simulink model "snb_bcxx"  (R2012b)
settings: Solver=FixedStepDiscrete  SolverMode=SingleTasking  StartTime=0.0  StopTime=10000  RelTol=1e-3
undefined symbols (not defined in the file): Down, pfb_coeff_gen_calc, Up
libraries: xbsIndex_r4 x19669, casper_library_misc x44, casper_library_delays x18, casper_library_communications x8, xps_library x3
(part 13 of 159)

== system snb_bcxx/pack ==
  note: Prevent transmission of data
      | before we have seen the first
      | sync
  rst : Inport
  sync_in : Inport  Port=2
  en : Inport  Port=3
  din : Inport  Port=4
  timestamp : Inport  Port=5
  flag : Inport  Port=6
  board_id : Inport  Port=7
  base_ip : Inport  Port=8
  base_port : Inport  Port=9
  AddSub : xbsIndex_r4/AddSub  mode=Addition  use_carryin=off  use_carryout=off  en=off  latency=1  precision=User Defined  arith_type=Unsigned  n_bits=32  bin_pt=0  quantization=Truncate  overflow=Wrap  dbl_ovrd=off  use_behavioral_HDL=off  hw_selection=Fabric  pipelined=off  block_type=addsub
  AddSub1 : xbsIndex_r4/AddSub  mode=Subtraction  use_carryin=off  use_carryout=off  en=on  latency=1  precision=Full  arith_type=Unsigned  n_bits=16  bin_pt=14  quantization=Truncate  overflow=Wrap  dbl_ovrd=off  use_behavioral_HDL=off  hw_selection=Fabric  pipelined=off  block_type=addsub
  Concat{,1..4} (5 alike) : xbsIndex_r4/Concat  num_inputs=2  dbl_ovrd=off  block_type=concat
  Concat10 : xbsIndex_r4/Concat  num_inputs=3  dbl_ovrd=off  block_type=concat
  Concat{5..8} (4 alike) : xbsIndex_r4/Concat  num_inputs=4  dbl_ovrd=off  block_type=concat
  Concat9 : xbsIndex_r4/Concat  num_inputs=3  dbl_ovrd=off  block_type=concat
  Constant : xbsIndex_r4/Constant  const=0  gui_display_data_type=Fixed-point  arith_type=Unsigned  n_bits=n_bits_packet - n_bits_inputs  bin_pt=0  preci_type=Single  exp_width=8  frac_width=24  explicit_period=on  period=1  equ=P=C  opselect=C  inp2=PCIN>>17  opr=+  inp1=P  carry=CIN  dbl_ovrd=off  block_type=constant
  Constant1 : xbsIndex_r4/Constant  const=0  gui_display_data_type=Fixed-point  arith_type=Unsigned  n_bits=2  bin_pt=0  preci_type=Single  exp_width=8  frac_width=24  explicit_period=on  period=1  equ=P=C  opselect=C  inp2=PCIN>>17  opr=+  inp1=P  carry=CIN  dbl_ovrd=off  block_type=constant
  Constant{7,10,13,16..19,39} (8 alike) : xbsIndex_r4/Constant  const=0  gui_display_data_type=Fixed-point  arith_type=Unsigned  n_bits=48  bin_pt=0  preci_type=Single  exp_width=8  frac_width=24  explicit_period=on  period=1  equ=P=C  opselect=C  inp2=PCIN>>17  opr=+  inp1=P  carry=CIN  dbl_ovrd=off  block_type=constant
  Constant{5,8,11,14} (4 alike) : xbsIndex_r4/Constant  const=1  gui_display_data_type=Fixed-point  arith_type=Unsigned  n_bits=48  bin_pt=0  preci_type=Single  exp_width=8  frac_width=24  explicit_period=on  period=1  equ=P=C  opselect=C  inp2=PCIN>>17  opr=+  inp1=P  carry=CIN  dbl_ovrd=off  block_type=constant
  Constant{6,9,12,15} (4 alike) : xbsIndex_r4/Constant  const=2^(n_bits_packet-n_bits_inputs)  gui_display_data_type=Fixed-point  arith_type=Unsigned  n_bits=48  bin_pt=0  preci_type=Single  exp_width=8  frac_width=24  explicit_period=on  period=1  equ=P=C  opselect=C  inp2=PCIN>>17  opr=+  inp1=P  carry=CIN  dbl_ovrd=off  block_type=constant
  Constant2 : xbsIndex_r4/Constant  const=1  gui_display_data_type=Fixed-point  arith_type=Unsigned  n_bits=2  bin_pt=0  preci_type=Single  exp_width=8  frac_width=24  explicit_period=on  period=1  equ=P=C  opselect=C  inp2=PCIN>>17  opr=+  inp1=P  carry=CIN  dbl_ovrd=off  block_type=constant
  Constant20 : xbsIndex_r4/Constant  const=0  gui_display_data_type=Fixed-point  arith_type=Unsigned  n_bits=n_bits_frequencies + n_bits_packet - n_bits_inputs  bin_pt=0  preci_type=Single  exp_width=8  frac_width=24  explicit_period=on  period=1  equ=P=C  opselect=C  inp2=PCIN>>17  opr=+  inp1=P  carry=CIN  dbl_ovrd=off  block_type=constant
  Constant3 : xbsIndex_r4/Constant  const=2  gui_display_data_type=Fixed-point  arith_type=Unsigned  n_bits=2  bin_pt=0  preci_type=Single  exp_width=8  frac_width=24  explicit_period=on  period=1  equ=P=C  opselect=C  inp2=PCIN>>17  opr=+  inp1=P  carry=CIN  dbl_ovrd=off  block_type=constant
  Constant4 : xbsIndex_r4/Constant  const=3  gui_display_data_type=Fixed-point  arith_type=Unsigned  n_bits=2  bin_pt=0  preci_type=Single  exp_width=8  frac_width=24  explicit_period=on  period=1  equ=P=C  opselect=C  inp2=PCIN>>17  opr=+  inp1=P  carry=CIN  dbl_ovrd=off  block_type=constant
  Convert{,2..9} (9 alike) : xbsIndex_r4/Convert  gui_display_data_type=Fixed-point  arith_type=Unsigned  n_bits=48  bin_pt=0  float_type=Single  exp_bits=8  fraction_bits=24  quantization=Truncate  overflow=Wrap  en=off  latency=0  dbl_ovrd=off  pipeline=off  block_type=convert
  Convert10 : xbsIndex_r4/Convert  gui_display_data_type=Fixed-point  arith_type=Unsigned  n_bits=32  bin_pt=0  float_type=Single  exp_bits=8  fraction_bits=24  quantization=Truncate  overflow=Wrap  en=off  latency=0  dbl_ovrd=off  pipeline=off  block_type=convert
  Delay{,16..20,27,31,33..34,37,39} (12 alike) : xbsIndex_r4/Delay  rst=off  infoeditControl=Selection of Reset will increase slice count due to use of real FFs and instead of SRLs  en=off  latency=1  dbl_ovrd=off  reg_retiming=on  block_type=delay
  Delay{1..15,21..26,28..30,32,35..36} (27 alike) : xbsIndex_r4/Delay  rst=off  infoeditControl=Selection of Reset will increase slice count due to use of real FFs and instead of SRLs  en=off  latency=2  dbl_ovrd=off  reg_retiming=on  block_type=delay
  Delay38 : xbsIndex_r4/Delay  rst=off  infoeditControl=Selection of Reset will increase slice count due to use of real FFs and instead of SRLs  en=off  latency=1  dbl_ovrd=off  reg_retiming=off  block_type=delay
  Logical{,1,6..8} (5 alike) : xbsIndex_r4/Logical  logical_function=AND  inputs=2  en=off  latency=0  precision=Full  arith_type=Unsigned  n_bits=16  bin_pt=0  align_bp=on  dbl_ovrd=off  block_type=logical
  Logical{2..5} (4 alike) : xbsIndex_r4/Logical  logical_function=AND  inputs=2  en=off  latency=1  precision=Full  arith_type=Unsigned  n_bits=16  bin_pt=0  align_bp=on  dbl_ovrd=off  block_type=logical
  Register : xbsIndex_r4/Register  init=0  rst=on  en=on  dbl_ovrd=off  block_type=register
  Register1 : xbsIndex_r4/Register  init=0  rst=on  en=on  dbl_ovrd=off  block_type=register
  Relational : xbsIndex_r4/Relational  mode=a=b  en=off  latency=0  dbl_ovrd=off  block_type=relational
  Relational1 : xbsIndex_r4/Relational  mode=a=b  en=off  latency=0  dbl_ovrd=off  block_type=relational
  Relational2 : xbsIndex_r4/Relational  mode=a!=b  en=off  latency=1  dbl_ovrd=off  block_type=relational
  Relational3 : xbsIndex_r4/Relational  mode=a!=b  en=off  latency=1  dbl_ovrd=off  block_type=relational
  Slice1 : xbsIndex_r4/Slice  nbits=n_bits_xengines - n_bits_xeng_per_ip  boolean_output=off  mode=Upper Bit Location + Width  bit1=0  base1=MSB of Input  bit0=0  base0=LSB of Input  dbl_ovrd=off  block_type=slice
  Slice2 : xbsIndex_r4/Slice  nbits=48  boolean_output=off  mode=Upper Bit Location + Width  bit1=0  base1=MSB of Input  bit0=0  base0=LSB of Input  dbl_ovrd=off  block_type=slice
  Slice3 : xbsIndex_r4/Slice  nbits=48  boolean_output=off  mode=Two Bit Locations  bit1=0  base1=MSB of Input  bit0=9+3  base0=LSB of Input  dbl_ovrd=off  block_type=slice
  Slice4 : xbsIndex_r4/Slice  nbits=4  boolean_output=off  mode=Lower Bit Location + Width  bit1=0  base1=MSB of Input  bit0=0  base0=LSB of Input  dbl_ovrd=off  block_type=slice
  Slice5 : xbsIndex_r4/Slice  nbits=48  boolean_output=off  mode=Two Bit Locations  bit1=0  base1=MSB of Input  bit0=9+3  base0=LSB of Input  dbl_ovrd=off  block_type=slice
  Slice6 : xbsIndex_r4/Slice  nbits=12  boolean_output=off  mode=Lower Bit Location + Width  bit1=0  base1=MSB of Input  bit0=0  base0=LSB of Input  dbl_ovrd=off  block_type=slice
  Terminator{15..18} (4 alike) : Terminator
  bus_expand : Subsystem  AncestorBlock=casper_library_flow_control/bus_expand  mask(bus_expand){mode=divisions of equal size, outputNum=4, outputWidth=64, outputBinaryPt=0, outputArithmeticType=0, show_format=off, outputToWorkspace=off, variablePrefix=out, outputToModelAsWell=on}
      mask prompts: outputNum "Number of outputs:"; outputWidth "Output width:"; outputBinaryPt "Output binary point position:"; outputArithmeticType "Output arithmetic type (ufix=0, fix=1, bool=2):"; show_format "Print format string?"; outputToWorkspace "Output to workspace?"; variablePrefix "Variable name prefix:"; outputToModelAsWell "Output to model as well?"
      mask help:
      | Expands a 'bus' made using a bus_create or Xilinx
      | concat block.
      | The input will be divided into the specified number
      | of outputs with the specified arithmetic types.
      | Divisions are made from most significant bit.
      mask init: same as snb_bcxx/bus_expand10
      settings: AttributesFormatString=4 outputs
      mask TypeOptions mode: divisions of equal size | divisions of arbitrary size
      mask Callback mode: bus_expand_callback();
      mask Callback outputWidth: bus_expand_callback();
      mask Callback outputToWorkspace: bus_expand_callback();
  bus_expand1 : Subsystem  AncestorBlock=casper_library_flow_control/bus_expand  mask(bus_expand){mode=divisions of equal size, outputNum=4, outputWidth=1, outputBinaryPt=0, outputArithmeticType=0, show_format=off, outputToWorkspace=off, variablePrefix=out, outputToModelAsWell=on}
      mask prompts: outputNum "Number of outputs:"; outputWidth "Output width:"; outputBinaryPt "Output binary point position:"; outputArithmeticType "Output arithmetic type (ufix=0, fix=1, bool=2):"; show_format "Print format string?"; outputToWorkspace "Output to workspace?"; variablePrefix "Variable name prefix:"; outputToModelAsWell "Output to model as well?"
      mask help:
      | Expands a 'bus' made using a bus_create or Xilinx
      | concat block.
      | The input will be divided into the specified number
      | of outputs with the specified arithmetic types.
      | Divisions are made from most significant bit.
      mask init: same as snb_bcxx/bus_expand10
      settings: AttributesFormatString=4 outputs
      mask TypeOptions mode: divisions of equal size | divisions of arbitrary size
      mask Callback mode: bus_expand_callback();
      mask Callback outputWidth: bus_expand_callback();
      mask Callback outputToWorkspace: bus_expand_callback();
  bus_expand2 : Subsystem  AncestorBlock=casper_library_flow_control/bus_expand  mask(bus_expand){mode=divisions of equal size, outputNum=4, outputWidth=16, outputBinaryPt=0, outputArithmeticType=0, show_format=off, outputToWorkspace=off, variablePrefix=out, outputToModelAsWell=on}
      mask prompts: outputNum "Number of outputs:"; outputWidth "Output width:"; outputBinaryPt "Output binary point position:"; outputArithmeticType "Output arithmetic type (ufix=0, fix=1, bool=2):"; show_format "Print format string?"; outputToWorkspace "Output to workspace?"; variablePrefix "Variable name prefix:"; outputToModelAsWell "Output to model as well?"
      mask help:
      | Expands a 'bus' made using a bus_create or Xilinx
      | concat block.
      | The input will be divided into the specified number
      | of outputs with the specified arithmetic types.
      | Divisions are made from most significant bit.
      mask init: same as snb_bcxx/bus_expand10
      settings: AttributesFormatString=4 outputs
      mask TypeOptions mode: divisions of equal size | divisions of arbitrary size
      mask Callback mode: bus_expand_callback();
      mask Callback outputWidth: bus_expand_callback();
      mask Callback outputToWorkspace: bus_expand_callback();
  count : xbsIndex_r4/Counter  cnt_type=Free Running  cnt_to=Inf  operation=Up  start_count=0  cnt_by_val=1  arith_type=Unsigned  n_bits=n_bits_frequencies + n_bits_packet - n_bits_inputs  bin_pt=0  load_pin=off  rst=on  en=on  explicit_period=on  period=1  dbl_ovrd=off  use_behavioral_HDL=off  implementation=Fabric  block_type=counter
  count1 : xbsIndex_r4/Counter  cnt_type=Free Running  cnt_to=Inf  operation=Up  start_count=0  cnt_by_val=1  arith_type=Unsigned  n_bits=n_bits_xengines  bin_pt=0  load_pin=off  rst=on  en=on  explicit_period=on  period=1  dbl_ovrd=off  use_behavioral_HDL=off  implementation=Fabric  block_type=counter
  divisions : xbsIndex_r4/Slice  nbits=n_bits_frequencies - n_bits_xengines  boolean_output=off  mode=Upper Bit Location + Width  bit1=0  base1=MSB of Input  bit0=0  base0=LSB of Input  dbl_ovrd=off  block_type=slice
  expected_diff : xbsIndex_r4/Constant  const=2^9  gui_display_data_type=Fixed-point  arith_type=Unsigned  n_bits=10  bin_pt=0  preci_type=Single  exp_width=8  frac_width=24  explicit_period=on  period=1  equ=P=C  opselect=C  inp2=PCIN>>17  opr=+  inp1=P  carry=CIN  dbl_ovrd=off  block_type=constant
  frequency : xbsIndex_r4/Slice  nbits=n_bits_frequencies  boolean_output=off  mode=Upper Bit Location + Width  bit1=0  base1=MSB of Input  bit0=0  base0=LSB of Input  dbl_ovrd=off  block_type=slice
  hdra_5 : xbsIndex_r4/Assert  assert_type=on  type_source=Explicitly  gui_display_data_type=Fixed-point  arith_type=Unsigned  n_bits=48  bin_pt=0  preci_type=Single  exp_width=8  frac_width=24  assert_rate=off  rate_source=Explicitly  period=1  output_port=on  block_type=assert
  pipeline1 : Subsystem  AncestorBlock=casper_library_delays/pipeline  mask(pipeline){latency=2}
      mask help:
      | An explicitly laid-out delay line to avoid mapping to SRL16s
      | for use in pipelining to help achieve timing closure.
      mask init:
      | pipeline_init(gcb,'latency',latency);
      settings: AttributesFormatString=Latency = %<latency>
      mask Display:
      | port_label('input', 1, 'd');
      | port_label('output', 1, 'q');
      | disp(['Z^-', num2str(latency)]);
  pipeline2 : Subsystem  AncestorBlock=casper_library_delays/pipeline  mask(pipeline){latency=1}
      mask help:
      | An explicitly laid-out delay line to avoid mapping to SRL16s
      | for use in pipelining to help achieve timing closure.
      mask init:
      | pipeline_init(gcb,'latency',latency);
      settings: AttributesFormatString=Latency = %<latency>
      mask Display:
      | port_label('input', 1, 'd');
      | port_label('output', 1, 'q');
      | disp(['Z^-', num2str(latency)]);
  pipeline3 : Subsystem  AncestorBlock=casper_library_delays/pipeline  mask(pipeline){latency=2}
      mask help:
      | An explicitly laid-out delay line to avoid mapping to SRL16s
      | for use in pipelining to help achieve timing closure.
      mask init:
      | pipeline_init(gcb,'latency',latency);
      settings: AttributesFormatString=Latency = %<latency>
      mask Display:
      | port_label('input', 1, 'd');
      | port_label('output', 1, 'q');
      | disp(['Z^-', num2str(latency)]);
  pipeline4 : Subsystem  AncestorBlock=casper_library_delays/pipeline  mask(pipeline){latency=2}
      mask help:
      | An explicitly laid-out delay line to avoid mapping to SRL16s
      | for use in pipelining to help achieve timing closure.
      mask init:
      | pipeline_init(gcb,'latency',latency);
      settings: AttributesFormatString=Latency = %<latency>
      mask Display:
      | port_label('input', 1, 'd');
      | port_label('output', 1, 'q');
      | disp(['Z^-', num2str(latency)]);
  pipeline5 : Subsystem  AncestorBlock=casper_library_delays/pipeline  mask(pipeline){latency=2}
      mask help:
      | An explicitly laid-out delay line to avoid mapping to SRL16s
      | for use in pipelining to help achieve timing closure.
      mask init:
      | pipeline_init(gcb,'latency',latency);
      settings: AttributesFormatString=Latency = %<latency>
      mask Display:
      | port_label('input', 1, 'd');
      | port_label('output', 1, 'q');
      | disp(['Z^-', num2str(latency)]);
  pipeline50 : Subsystem  AncestorBlock=casper_library_delays/pipeline  mask(pipeline){latency=2}
      mask help:
      | An explicitly laid-out delay line to avoid mapping to SRL16s
      | for use in pipelining to help achieve timing closure.
      mask init:
      | pipeline_init(gcb,'latency',latency);
      settings: AttributesFormatString=Latency = %<latency>
      mask Display:
      | port_label('input', 1, 'd');
      | port_label('output', 1, 'q');
      | disp(['Z^-', num2str(latency)]);
  pipeline6 : Subsystem  AncestorBlock=casper_library_delays/pipeline  mask(pipeline){latency=2}
      mask help:
      | An explicitly laid-out delay line to avoid mapping to SRL16s
      | for use in pipelining to help achieve timing closure.
      mask init:
      | pipeline_init(gcb,'latency',latency);
      settings: AttributesFormatString=Latency = %<latency>
      mask Display:
      | port_label('input', 1, 'd');
      | port_label('output', 1, 'q');
      | disp(['Z^-', num2str(latency)]);
  pipeline7 : Subsystem  AncestorBlock=casper_library_delays/pipeline  mask(pipeline){latency=2}
      mask help:
      | An explicitly laid-out delay line to avoid mapping to SRL16s
      | for use in pipelining to help achieve timing closure.
      mask init:
      | pipeline_init(gcb,'latency',latency);
      settings: AttributesFormatString=Latency = %<latency>
      mask Display:
      | port_label('input', 1, 'd');
      | port_label('output', 1, 'q');
      | disp(['Z^-', num2str(latency)]);
  sample_count : xbsIndex_r4/Slice  nbits=n_bits_packet - n_bits_inputs  boolean_output=off  mode=Lower Bit Location + Width  bit1=0  base1=MSB of Input  bit0=0  base0=LSB of Input  dbl_ovrd=off  block_type=slice
  select_we : xbsIndex_r4/Mux  inputs=2  en=off  latency=0  precision=Full  arith_type=Unsigned  n_bits=16  bin_pt=14  quantization=Truncate  overflow=Wrap  dbl_ovrd=off  block_type=mux
  spead_pack : Subsystem  Tag=casper:spead_pack  AncestorBlock=casper_library_communications/spead_pack  mask(pkt_pack_mask){max_pkt_len_bits=10, header_ids=0x1600, 0x4101, 0x4102, 0x4103, header_ind_ids=0x4300, spead_msw=64, spead_lsw=48, spead_version=4, bytes_per_word=8}
      mask prompts: max_pkt_len_bits "Max pkt length, 2^? 64-bit words"; header_ids "SPEAD direct address IDs (decimal)"; header_ind_ids "SPEAD indirect address IDs (decimal)"; spead_msw "SPEAD Flavour (MSw)"; spead_lsw "SPEAD Flavour (LSw)"; spead_version "SPEAD version"; bytes_per_word "Word size, in bytes"
      mask help:
      | This block generates SPEAD-compliant packets from a datastream.
      |
      | Packets are created with a fixed header followed by a number of 64-bit items.
      |
      | Requires a 64-bit data stream.
      |
      | The data_ready signal is one cycle BEFORE valid data! Does not have to be with a valid signal either.
      mask init:
      | if floor(log2(bytes_per_word)) ~= log2(bytes_per_word)
      |     error('Bytes per word should be a power of two.');
      | end
      | 
      | spead_pack_init(gcb)
  spead_pack1 : Subsystem  Tag=casper:spead_pack  AncestorBlock=casper_library_communications/spead_pack  mask(pkt_pack_mask){max_pkt_len_bits=10, header_ids=0x1600, 0x4101, 0x4102, 0x4103, header_ind_ids=0x4300, spead_msw=64, spead_lsw=48, spead_version=4, bytes_per_word=8}
      mask prompts: max_pkt_len_bits "Max pkt length, 2^? 64-bit words"; header_ids "SPEAD direct address IDs (decimal)"; header_ind_ids "SPEAD indirect address IDs (decimal)"; spead_msw "SPEAD Flavour (MSw)"; spead_lsw "SPEAD Flavour (LSw)"; spead_version "SPEAD version"; bytes_per_word "Word size, in bytes"
      mask help:
      | This block generates SPEAD-compliant packets from a datastream.
      |
      | Packets are created with a fixed header followed by a number of 64-bit items.
      |
      | Requires a 64-bit data stream.
      |
      | The data_ready signal is one cycle BEFORE valid data! Does not have to be with a valid signal either.
      mask init:
      | if floor(log2(bytes_per_word)) ~= log2(bytes_per_word)
      |     error('Bytes per word should be a power of two.');
      | end
      | 
      | spead_pack_init(gcb)
  spead_pack2 : Subsystem  Tag=casper:spead_pack  AncestorBlock=casper_library_communications/spead_pack  mask(pkt_pack_mask){max_pkt_len_bits=10, header_ids=0x1600, 0x4101, 0x4102, 0x4103, header_ind_ids=0x4300, spead_msw=64, spead_lsw=48, spead_version=4, bytes_per_word=8}
      mask prompts: max_pkt_len_bits "Max pkt length, 2^? 64-bit words"; header_ids "SPEAD direct address IDs (decimal)"; header_ind_ids "SPEAD indirect address IDs (decimal)"; spead_msw "SPEAD Flavour (MSw)"; spead_lsw "SPEAD Flavour (LSw)"; spead_version "SPEAD version"; bytes_per_word "Word size, in bytes"
      mask help:
      | This block generates SPEAD-compliant packets from a datastream.
      |
      | Packets are created with a fixed header followed by a number of 64-bit items.
      |
      | Requires a 64-bit data stream.
      |
      | The data_ready signal is one cycle BEFORE valid data! Does not have to be with a valid signal either.
      mask init:
      | if floor(log2(bytes_per_word)) ~= log2(bytes_per_word)
      |     error('Bytes per word should be a power of two.');
      | end
      | 
      | spead_pack_init(gcb)
  spead_pack3 : Subsystem  Tag=casper:spead_pack  AncestorBlock=casper_library_communications/spead_pack  mask(pkt_pack_mask){max_pkt_len_bits=10, header_ids=0x1600, 0x4101, 0x4102, 0x4103, header_ind_ids=0x4300, spead_msw=64, spead_lsw=48, spead_version=4, bytes_per_word=8}
      mask prompts: max_pkt_len_bits "Max pkt length, 2^? 64-bit words"; header_ids "SPEAD direct address IDs (decimal)"; header_ind_ids "SPEAD indirect address IDs (decimal)"; spead_msw "SPEAD Flavour (MSw)"; spead_lsw "SPEAD Flavour (LSw)"; spead_version "SPEAD version"; bytes_per_word "Word size, in bytes"
      mask help:
      | This block generates SPEAD-compliant packets from a datastream.
      |
      | Packets are created with a fixed header followed by a number of 64-bit items.
      |
      | Requires a 64-bit data stream.
      |
      | The data_ready signal is one cycle BEFORE valid data! Does not have to be with a valid signal either.
      mask init:
      | if floor(log2(bytes_per_word)) ~= log2(bytes_per_word)
      |     error('Bytes per word should be a power of two.');
      | end
      | 
      | spead_pack_init(gcb)
  wintime : xbsIndex_r4/Register  init=0  rst=off  en=on  dbl_ovrd=off  block_type=register
  wintime_old : xbsIndex_r4/Register  init=0  rst=off  en=on  dbl_ovrd=off  block_type=register
  xengines : xbsIndex_r4/Slice  nbits=n_bits_xengines  boolean_output=off  mode=Lower Bit Location + Width  bit1=0  base1=MSB of Input  bit0=0  base0=LSB of Input  dbl_ovrd=off  block_type=slice
  dout : Outport
  dvalid : Outport  Port=2
  eof : Outport  Port=3
  overflow : Outport  Port=4
  destination_ip : Outport  Port=5
  destination_port : Outport  Port=6
  wintime_snap : Outport  Port=7
  wintime_error : Outport  Port=8
  wintime_sp_error : Outport  Port=9
  wires:
  Slice1/1 -> Convert10/1
  Convert10/1 -> AddSub/2
  AddSub/1 -> destination_ip/1  "ip"
  count1/1 -> Slice1/1
  Delay19/1 -> destination_port/1  "port"
  base_port/1 -> Delay19/1
  Delay18/1 -> eof/1
  Delay16/1 -> dvalid/1
  Delay17/1 -> dout/1
  base_ip/1 -> AddSub/1
  Concat8/1 -> Delay20/1
  Concat7/1 -> Delay18/1
  Concat6/1 -> Delay16/1
  Concat5/1 -> Delay17/1
  Concat4/1 -> Delay15/1
  Delay15/1 -> Convert4/1
  Constant4/1 -> Concat4/2
  Delay14/1 -> Convert9/1
  Delay9/1 -> Convert5/1
  Concat3/1 -> Delay9/1
  Constant3/1 -> Concat3/2
  Delay10/1 -> Convert8/1
  Delay12/1 -> Convert6/1
  Delay11/1 -> Convert7/1
  Concat2/1 -> Delay12/1
  Concat1/1 -> Concat4/1, Concat3/1, Concat2/1, Concat/1
  Constant2/1 -> Concat2/2
  flag/1 -> bus_expand1/1(bus_in)
  divisions/1 -> Concat1/2
  xengines/1 -> Concat1/1
  frequency/1 -> xengines/1, divisions/1  "fchan"
  Concat/1 -> Delay6/1
  Constant1/1 -> Concat/2
  Logical1/1 -> count/2, Logical8/2, select_we/3, Logical/2, Delay1/1  "en2"
  en/1 -> Logical1/2  "en"
  Register/1 -> Logical1/1  "arm"
  rst/1 -> Register/2  "rst"
  sync_in/1 -> count/1, [sync], Register/1, Register/3  "sync"
  Delay2/1 -> spead_pack/3(data64)
  Delay6/1 -> Convert/1
  Delay5/1 -> Convert3/1
  Delay4/1 -> Convert2/1
  Delay3/1 -> Slice2/1
  Delay1/1 -> [d64_valid], spead_pack/2(data64_valid)  "dvalid"
  Delay/1 -> [d64_ready], spead_pack/1(data64_ready)  "dready"
  Logical/1 -> Delay/1
  Relational/1 -> Logical/1
  Constant/1 -> Relational/2
  sample_count/1 -> Relational/1  "sample_cnt"
  din/1 -> bus_expand/1(bus_in)
  board_id/1 -> Delay4/1
  Convert2/1 -> [hdr2], spead_pack/9(hdr6_0x4101_DIR)
  Slice2/1 -> spead_pack/8(hdr5_0x1600_DIR), spead_pack/4(hdr_heap_id), [hdr1]  "time"
  count/1 -> sample_count/1, Relational1/2, frequency/1  "fcount"
  Delay20/1 -> overflow/1
  Constant5/1 -> spead_pack/5(hdr_heap_size)
  Constant39/1 -> spead_pack/6(hdr_heap_offset)
  Constant6/1 -> spead_pack/7(hdr_pkt_len_words)
  Constant8/1 -> spead_pack1/5(hdr_heap_size)
  Constant7/1 -> spead_pack1/6(hdr_heap_offset)
  Constant9/1 -> spead_pack1/7(hdr_pkt_len_words)
  Convert3/1 -> spead_pack/10(hdr7_0x4102_DIR)
  Convert/1 -> [x4103_0], spead_pack/11(hdr8_0x4103_DIR)
  Constant11/1 -> spead_pack2/5(hdr_heap_size)
  Constant10/1 -> spead_pack2/6(hdr_heap_offset)
  Constant12/1 -> spead_pack2/7(hdr_pkt_len_words)
  Constant14/1 -> spead_pack3/5(hdr_heap_size)
  Constant13/1 -> spead_pack3/6(hdr_heap_offset)
  Constant15/1 -> spead_pack3/7(hdr_pkt_len_words)
  [d64_ready] -> spead_pack1/1(data64_ready)
  [d64_valid] -> spead_pack1/2(data64_valid)
  [hdr1] -> spead_pack1/8(hdr5_0x1600_DIR), spead_pack1/4(hdr_heap_id)
  Delay7/1 -> spead_pack1/3(data64)
  [d64_ready] -> spead_pack2/1(data64_ready)
  [d64_valid] -> spead_pack2/2(data64_valid)
  [hdr1] -> spead_pack2/8(hdr5_0x1600_DIR), spead_pack2/4(hdr_heap_id)
  Delay8/1 -> spead_pack2/3(data64)
  [d64_ready] -> spead_pack3/1(data64_ready)
  [d64_valid] -> spead_pack3/2(data64_valid)
  [hdr1] -> spead_pack3/8(hdr5_0x1600_DIR), spead_pack3/4(hdr_heap_id)
  Delay13/1 -> spead_pack3/3(data64)
  [hdr2] -> spead_pack1/9(hdr6_0x4101_DIR)
  Convert7/1 -> spead_pack1/10(hdr7_0x4102_DIR)
  Convert6/1 -> spead_pack1/11(hdr8_0x4103_DIR)
  Convert5/1 -> spead_pack2/11(hdr8_0x4103_DIR)
  Convert8/1 -> spead_pack2/10(hdr7_0x4102_DIR)
  [hdr2] -> spead_pack2/9(hdr6_0x4101_DIR)
  Convert9/1 -> spead_pack3/10(hdr7_0x4102_DIR)
  Convert4/1 -> spead_pack3/11(hdr8_0x4103_DIR)
  [hdr2] -> spead_pack3/9(hdr6_0x4101_DIR)
  [d64_3] -> Concat5/4
  [d64_2] -> Concat5/3
  [d64_1] -> Concat5/2
  [d64_0] -> Concat5/1
  [v64_3] -> Concat6/4
  [v64_0] -> Concat6/1
  [v64_2] -> Concat6/3
  [v64_1] -> Concat6/2
  [e64_0] -> Concat7/1
  [o64_0] -> Concat8/1
  [e64_1] -> Concat7/2
  [e64_3] -> Concat7/4
  [e64_2] -> Concat7/3
  [o64_1] -> Concat8/2
  [o64_3] -> Concat8/4
  [o64_2] -> Concat8/3
  bus_expand/1(msb_out4) -> [din_0]
  bus_expand/2(out3) -> [din_1]
  bus_expand/3(out2) -> [din_2]
  bus_expand/4(lsb_out1) -> [din_3]
  [din_0] -> Delay2/1
  [din_1] -> Delay7/1
  [din_2] -> Delay8/1
  [din_3] -> Delay13/1
  bus_expand1/1(msb_out4) -> [flags_0]
  bus_expand1/2(out3) -> [flags_1]
  bus_expand1/3(out2) -> [flags_2]
  bus_expand1/4(lsb_out1) -> [flags_3]
  [flags_0] -> Delay5/1
  [flags_1] -> Delay11/1
  [flags_2] -> Delay10/1
  [flags_3] -> Delay14/1
  hdra_5/1 -> [time48], Delay3/1
  timestamp/1 -> hdra_5/1  "time"
  bus_expand2/4(lsb_out1) -> Terminator18/1  "f3"
  bus_expand2/3(out2) -> Terminator17/1  "f2"
  bus_expand2/2(out3) -> Terminator16/1  "f1"
  bus_expand2/1(msb_out4) -> Terminator15/1  "f0"
  Delay23/1 -> [o64_0]  "of64_0"
  Delay22/1 -> [v64_0]  "valid64_0"
  Delay21/1 -> [d64_0], bus_expand2/1(bus_in)  "data64_0"
  Logical3/1 -> [e64_pre], Delay34/1  "eof64_pre"
  Delay34/1 -> [e64_0]  "eof64_0"
  Logical6/1 -> count1/2  "next_ip"
  [e64_pre] -> Delay33/1, Register1/3, Register1/1
  Register1/1 -> Logical6/1  "ip_arm"
  [sync] -> Register1/2
  Delay33/1 -> Logical6/2
  [sync] -> count1/1
  spead_pack/1(data_out) -> Delay21/1
  spead_pack/2(valid_out) -> Logical3/1, Delay22/1
  spead_pack/3(eof) -> Logical3/2
  spead_pack/4(data_overflow) -> Delay23/1
  Constant16/1 -> spead_pack/12(hdr9_0x4300)
  Delay26/1 -> [o64_1]  "of64_0"
  Delay25/1 -> [v64_1]  "valid64_0"
  Delay24/1 -> [d64_1]  "data64_0"
  Logical2/1 -> Delay27/1  "eof64_pre"
  Delay27/1 -> [e64_1]  "eof64_0"
  spead_pack1/1(data_out) -> Delay24/1
  spead_pack1/2(valid_out) -> Logical2/1, Delay25/1
  spead_pack1/3(eof) -> Logical2/2
  spead_pack1/4(data_overflow) -> Delay26/1
  Constant17/1 -> spead_pack1/12(hdr9_0x4300)
  Delay30/1 -> [o64_2]  "of64_0"
  Delay29/1 -> [v64_2]  "valid64_0"
  Delay28/1 -> [d64_2]  "data64_0"
  Logical4/1 -> Delay31/1  "eof64_pre"
  Delay31/1 -> [e64_2]  "eof64_0"
  spead_pack2/1(data_out) -> Delay28/1
  spead_pack2/2(valid_out) -> Logical4/1, Delay29/1
  spead_pack2/3(eof) -> Logical4/2
  spead_pack2/4(data_overflow) -> Delay30/1
  Constant18/1 -> spead_pack2/12(hdr9_0x4300)
  Delay36/1 -> [o64_3]  "of64_0"
  Delay35/1 -> [v64_3]  "valid64_0"
  Delay32/1 -> [d64_3]  "data64_0"
  Logical5/1 -> Delay37/1  "eof64_pre"
  Delay37/1 -> [e64_3]  "eof64_0"
  spead_pack3/1(data_out) -> Delay32/1
  spead_pack3/2(valid_out) -> Logical5/1, Delay35/1
  spead_pack3/3(eof) -> Logical5/2
  spead_pack3/4(data_overflow) -> Delay36/1
  Constant19/1 -> spead_pack3/12(hdr9_0x4300)
  Constant20/1 -> Relational1/1
  [time48] -> Slice3/1
  Logical8/1 -> pipeline2/1(d), select_we/2, pipeline4/1(d), pipeline5/1(d)  "window_start"
  wintime/1 -> AddSub1/1, Relational3/1, wintime_old/1  "window_time"
  Delay38/1 -> AddSub1/3
  AddSub1/1 -> Relational2/2  "diff"
  expected_diff/1 -> Relational2/1
  Relational2/1 -> wintime_error/1  "differror"
  wintime_old/1 -> AddSub1/2  "window_time_old"
  Slice3/1 -> Concat10/1, pipeline3/1(d)
  [hdr1] -> pipeline6/1(d)
  Slice5/1 -> Relational3/2
  Relational3/1 -> Logical7/1
  Logical7/1 -> wintime_sp_error/1
  [d64_valid] -> pipeline7/1(d)
  Delay39/1 -> Logical7/2
  Relational1/1 -> Logical8/1  "window_start"
  Concat9/1 -> wintime_snap/1
  [hdr2] -> Slice4/1
  [x4103_0] -> Slice6/1
  select_we/1 -> pipeline1/1(d)
  Concat10/1 -> pipeline50/1(d)
  Slice4/1 -> Concat10/2
  Slice6/1 -> Concat10/3
  [wintime_snap_wesel] -> select_we/1
  pipeline50/1(q) -> Concat9/1
  pipeline1/1(q) -> Concat9/2
  pipeline2/1(q) -> Concat9/3
  pipeline3/1(q) -> wintime/1
  pipeline4/1(q) -> wintime/2
  pipeline5/1(q) -> wintime_old/2, Delay38/1
  pipeline6/1(q) -> Slice5/1
  pipeline7/1(q) -> Delay39/1

== system snb_bcxx/pfb_fft ==
  sync : Inport
  dv : Inport  Port=2
  pol0 : Inport  Port=3
  pol1 : Inport  Port=4
  shift : Inport  Port=5
  Convert4 : xbsIndex_r4/Convert  gui_display_data_type=Boolean  arith_type=Boolean  n_bits=18  bin_pt=17  float_type=Single  exp_bits=8  fraction_bits=24  quantization=Truncate  overflow=Wrap  en=off  latency=0  dbl_ovrd=off  pipeline=off  block_type=convert
  a0p0_1st_shift : Subsystem  mask{shift=1, latency=1}
      mask prompts: shift "Number bits to shift right by"; latency "Shift latency"
  c_to_ri : casper_library_misc/c_to_ri  n_bits=18  bin_pt=17
  c_to_ri1 : casper_library_misc/c_to_ri  n_bits=18  bin_pt=17
  fft_biplex : Subsystem  AncestorBlock=casper_library_ffts/fft_biplex  mask(fft_biplex){n_streams=1, n_inputs=1, FFTSize=13, input_bit_width=18, bin_pt_in=17, coeff_bit_width=18, async=on, add_latency=1, mult_latency=2, bram_latency=2, conv_latency=1, quantization=Round  (unbiased: +/- Inf), overflow=Saturate, coeffs_bit_limit=8, delays_bit_limit=8, coeff_sharing=on, coeff_decimation=on, max_fanout=4, mult_spec=2, bitgrowth=off, max_bits=18, hardcode_shifts=off, shift_schedule=[1                                      1], dsp48_adders=off}
      mask prompts: n_streams "Number simultaneous streams"; n_inputs "Number simultaneous inputs (2*?)"; FFTSize "Size of FFT: (2^? pts)"; input_bit_width "Input bit width"; bin_pt_in "input binary point"; coeff_bit_width "Coefficient Bit Width"; async "Asynchronous operation"; add_latency "Add Latency"; mult_latency "Mult Latency"; bram_latency "BRAM Latency"; conv_latency "Convert latency"; quantization "Quantization Behavior"; overflow "Overflow Behavior"; coeffs_bit_limit "Number bits above which to store stage's coefficients in BRAM (2^? bits)"; delays_bit_limit "Number bits above which to implent stage's delays in BRAM (2^? bits)"; coeff_sharing "BRAM sharing in coeff storage"; coeff_decimation "Store a fraction of coeff factors where useful"; max_fanout "Maximum fanout"; mult_spec "Multiplier impl. (0=core, 1=embedded, 2=behavioural) (left=1st stage, or just one value)"; bitgrowth "Bit growth instead of shift"; max_bits "Maximum bits to grow to"; hardcode_shifts "Hardcode shift schedule"; shift_schedule "Shift schedule"; dsp48_adders "Use DSP48s for adders"
      mask help: FFT internal block.
      mask init:
      | fft_biplex_init(gcb, ...
      |     'n_streams', n_streams, ...
      |     'n_inputs', n_inputs, ...
      |     'FFTSize', FFTSize, ...
      |     'input_bit_width', input_bit_width, ...
      |     'bin_pt_in', bin_pt_in, ...
      |     'coeff_bit_width', coeff_bit_width, ...
      |     'async', async, ...
      |     'add_latency', add_latency, ...
      |     'mult_latency', mult_latency, ...
      |     'bram_latency', bram_latency, ...
      |     'conv_latency', conv_latency, ...
      |     'quantization', quantization, ...
      |     'overflow', overflow, ...
      |     'coeffs_bit_limit', coeffs_bit_limit, ...
      |     'delays_bit_limit', delays_bit_limit, ...
      |     'coeff_sharing', coeff_sharing, ...
      |     'coeff_decimation', coeff_decimation, ...
      |     'max_fanout', max_fanout, ...
      |     'mult_spec', mult_spec, ...
      |     'bitgrowth', bitgrowth, ...
      |     'max_bits', max_bits, ...
      |     'hardcode_shifts', hardcode_shifts, ...
      |     'shift_schedule', shift_schedule, ...
      |     'dsp48_adders', dsp48_adders);
      settings: AttributesFormatString=13 stages
      mask TypeOptions quantization: Truncate | Round  (unbiased: +/- Inf) | Round  (unbiased: Even Values)
      mask TypeOptions overflow: Wrap | Saturate | Error
      mask Callback hardcode_shifts:
      | hardcode_shifts = get_param(gcb, 'hardcode_shifts');
      | set_param_state(gcb, 'shift_schedule', hardcode_shifts);
      mask Callback dsp48_adders: fft_callback_dsp48_adders(gcb);
  pfb_fir_generic : Subsystem  Tag=casper:pfb_fir_generic  AncestorBlock=casper_library_pfbs/pfb_fir_generic  mask(pfb_fir_generic){n_streams=2, PFBSize=13, TotalTaps=8, WindowType=hamming, n_inputs=0, BitWidthIn=18, BitWidthOut=18, CoeffBitWidth=18, complex=on, async=on, add_latency=2, mult_latency=3, bram_latency=8, fan_latency=9, conv_latency=2, quantization=Round  (unbiased: Even Values), fwidth=1, coeffs_bram_optimization=Speed, delays_bram_optimization=Speed}
      mask prompts: n_streams "Number input streams?"; PFBSize "Size of PFB: (2^? pnts)"; TotalTaps "Total Number of Taps:"; WindowType "Windowing Function:"; n_inputs "Number of Simultaneous Inputs: (2^?)"; BitWidthIn "Input Bitwidth:"; BitWidthOut "Output Bitwidth:"; CoeffBitWidth "Coefficient Bitwidth:"; complex "Complex data inputs"; async "Asynchronous operation"; add_latency "Add Latency"; mult_latency "Mult Latency"; bram_latency "BRAM Latency"; fan_latency "Fanout Latency"; conv_latency "Convert latency"; quantization "Quantization Behavior"; fwidth "Bin Width Scaling (normal=1)"; coeffs_bram_optimization "Coefficient BRAMs optimization"; delays_bram_optimization "Delay BRAMs optimization"
      mask init:
      | pfb_fir_generic_init(gcb, ...
      |     'n_streams', n_streams, ...
      |     'PFBSize', PFBSize, ...
      |     'TotalTaps', TotalTaps, ...
      |     'WindowType', WindowType, ...
      |     'n_inputs', n_inputs, ...
      |     'complex', complex, ...
      |     'BitWidthIn', BitWidthIn, ...
      |     'BitWidthOut', BitWidthOut, ...
      |     'CoeffBitWidth', CoeffBitWidth, ...
      |     'async', async, ...
      |     'add_latency', add_latency, ...
      |     'mult_latency', mult_latency, ...
      |     'bram_latency', bram_latency, ...
      |     'fan_latency', fan_latency, ...
      |     'conv_latency', conv_latency, ...
      |     'quantization', quantization, ...
      |     'fwidth', fwidth, ...
      |     'coeffs_bram_optimization', coeffs_bram_optimization, ...
      |     'delays_bram_optimization', delays_bram_optimization);
      mask Callback TotalTaps:
      | %num_taps = eval(get_param(gcb, 'TotalTaps'));
      | %old_vec = eval(get_param(gcb, 'mult_spec'));
      | 
      | %vec = 2.*ones(1,num_taps);
      | %old_size = length(old_vec);
      | 
      | %if(old_size <= num_taps),
      | %   new_size = old_size;
      | %else,
      | %    new_size = num_taps;
      | %end
      | 
      | %for n = 1:new_size, vec(n) = old_vec(n); end
      | %set_param(gcb, 'mult_spec', mat2str(vec));
      mask TypeOptions WindowType: bartlett | barthannwin | blackman | blackmanharris | bohamwin | chebwin | flattopwin | gausswin | hamming | hann | kaiser | nuttallwin | parzenwin | rectwin | tukeywin | triang | userwindow
      mask TypeOptions quantization: Truncate | Round  (unbiased: +/- Inf) | Round  (unbiased: Even Values)
      mask Callback fwidth:
      | %num_taps = eval(get_param(gcb, 'TotalTaps'));
      | %old_vec = eval(get_param(gcb, 'mult_spec'));
      | 
      | %vec = 2.*ones(1,num_taps);
      | %old_size = length(old_vec);
      | 
      | %if(old_size <= num_taps),
      | %    new_size = old_size;
      | %else,
      | %    new_size = num_taps;
      | %end
      | 
      | %for n = 1:new_size, vec(n) = old_vec(n); end
      | %set_param(gcb, 'mult_spec', mat2str(vec));
      mask TypeOptions coeffs_bram_optimization: Area | Speed
      mask TypeOptions delays_bram_optimization: Area | Speed
  pipeline1 : Subsystem  AncestorBlock=casper_library_delays/pipeline  mask(pipeline){latency=2}
      mask help:
      | An explicitly laid-out delay line to avoid mapping to SRL16s
      | for use in pipelining to help achieve timing closure.
      mask init:
      | pipeline_init(gcb,'latency',latency);
      settings: AttributesFormatString=Latency = %<latency>
      mask Display:
      | port_label('input', 1, 'd');
      | port_label('output', 1, 'q');
      | disp(['Z^-', num2str(latency)]);
  pipeline2 : Subsystem  AncestorBlock=casper_library_delays/pipeline  mask(pipeline){latency=2}
      mask help:
      | An explicitly laid-out delay line to avoid mapping to SRL16s
      | for use in pipelining to help achieve timing closure.
      mask init:
      | pipeline_init(gcb,'latency',latency);
      settings: AttributesFormatString=Latency = %<latency>
      mask Display:
      | port_label('input', 1, 'd');
      | port_label('output', 1, 'q');
      | disp(['Z^-', num2str(latency)]);
  pipeline3 : Subsystem  AncestorBlock=casper_library_delays/pipeline  mask(pipeline){latency=2}
      mask help:
      | An explicitly laid-out delay line to avoid mapping to SRL16s
      | for use in pipelining to help achieve timing closure.
      mask init:
      | pipeline_init(gcb,'latency',latency);
      settings: AttributesFormatString=Latency = %<latency>
      mask Display:
      | port_label('input', 1, 'd');
      | port_label('output', 1, 'q');
      | disp(['Z^-', num2str(latency)]);
  pipeline4 : Subsystem  AncestorBlock=casper_library_delays/pipeline  mask(pipeline){latency=3}
      mask help:
      | An explicitly laid-out delay line to avoid mapping to SRL16s
      | for use in pipelining to help achieve timing closure.
      mask init:
      | pipeline_init(gcb,'latency',latency);
      settings: AttributesFormatString=Latency = %<latency>
      mask Display:
      | port_label('input', 1, 'd');
      | port_label('output', 1, 'q');
      | disp(['Z^-', num2str(latency)]);
  pipeline5 : Subsystem  AncestorBlock=casper_library_delays/pipeline  mask(pipeline){latency=3}
      mask help:
      | An explicitly laid-out delay line to avoid mapping to SRL16s
      | for use in pipelining to help achieve timing closure.
      mask init:
      | pipeline_init(gcb,'latency',latency);
      settings: AttributesFormatString=Latency = %<latency>
      mask Display:
      | port_label('input', 1, 'd');
      | port_label('output', 1, 'q');
      | disp(['Z^-', num2str(latency)]);
  pipeline6 : Subsystem  AncestorBlock=casper_library_delays/pipeline  mask(pipeline){latency=3}
      mask help:
      | An explicitly laid-out delay line to avoid mapping to SRL16s
      | for use in pipelining to help achieve timing closure.
      mask init:
      | pipeline_init(gcb,'latency',latency);
      settings: AttributesFormatString=Latency = %<latency>
      mask Display:
      | port_label('input', 1, 'd');
      | port_label('output', 1, 'q');
      | disp(['Z^-', num2str(latency)]);
  pipeline7 : Subsystem  AncestorBlock=casper_library_delays/pipeline  mask(pipeline){latency=3}
      mask help:
      | An explicitly laid-out delay line to avoid mapping to SRL16s
      | for use in pipelining to help achieve timing closure.
      mask init:
      | pipeline_init(gcb,'latency',latency);
      settings: AttributesFormatString=Latency = %<latency>
      mask Display:
      | port_label('input', 1, 'd');
      | port_label('output', 1, 'q');
      | disp(['Z^-', num2str(latency)]);
  pipeline8 : Subsystem  AncestorBlock=casper_library_delays/pipeline  mask(pipeline){latency=3}
      mask help:
      | An explicitly laid-out delay line to avoid mapping to SRL16s
      | for use in pipelining to help achieve timing closure.
      mask init:
      | pipeline_init(gcb,'latency',latency);
      settings: AttributesFormatString=Latency = %<latency>
      mask Display:
      | port_label('input', 1, 'd');
      | port_label('output', 1, 'q');
      | disp(['Z^-', num2str(latency)]);
  pipeline81 : Subsystem  AncestorBlock=casper_library_delays/pipeline  mask(pipeline){latency=2}
      mask help:
      | An explicitly laid-out delay line to avoid mapping to SRL16s
      | for use in pipelining to help achieve timing closure.
      mask init:
      | pipeline_init(gcb,'latency',latency);
      settings: AttributesFormatString=Latency = %<latency>
      mask Display:
      | port_label('input', 1, 'd');
      | port_label('output', 1, 'q');
      | disp(['Z^-', num2str(latency)]);
  ri_to_c : casper_library_misc/ri_to_c
  ri_to_c1 : casper_library_misc/ri_to_c
  sync_out : Outport
  dv_out : Outport  Port=2
  pol0_out : Outport  Port=3
  pol1_out : Outport  Port=4
  of : Outport  Port=5
  wires:
  pol1/1 -> pfb_fir_generic/3(pol1_in0)
  pol0/1 -> pfb_fir_generic/2(pol0_in0)
  dv/1 -> pfb_fir_generic/4(en)
  pfb_fir_generic/4(dvalid) -> pipeline3/1(d)
  c_to_ri1/2 -> a0p0_1st_shift/5(din4)
  c_to_ri1/1 -> a0p0_1st_shift/4(din3)
  c_to_ri/2 -> a0p0_1st_shift/3(din2)
  c_to_ri/1 -> a0p0_1st_shift/2(din1)
  pfb_fir_generic/1(sync_out) -> pipeline81/1(d)
  pfb_fir_generic/2(pol0_out0) -> pipeline1/1(d)
  sync/1 -> pfb_fir_generic/1(sync)
  Convert4/1 -> of/1
  a0p0_1st_shift/3(dout1) -> ri_to_c/1
  a0p0_1st_shift/4(dout2) -> ri_to_c/2
  a0p0_1st_shift/5(dout3) -> ri_to_c1/1
  a0p0_1st_shift/6(dout4) -> ri_to_c1/2
  a0p0_1st_shift/1(sync_out) -> pipeline4/1(d)
  shift/1 -> pipeline5/1(d)
  a0p0_1st_shift/2(dvalid) -> pipeline8/1(d)
  ri_to_c/1 -> pipeline6/1(d)
  ri_to_c1/1 -> pipeline7/1(d)
  fft_biplex/1(sync_out) -> sync_out/1
  fft_biplex/5(dvalid) -> dv_out/1
  fft_biplex/2(pol00_out) -> pol0_out/1
  fft_biplex/3(pol01_out) -> pol1_out/1
  fft_biplex/4(of) -> Convert4/1
  pipeline81/1(q) -> a0p0_1st_shift/1(sync_in)
  pipeline1/1(q) -> c_to_ri/1
  pfb_fir_generic/3(pol1_out0) -> pipeline2/1(d)
  pipeline2/1(q) -> c_to_ri1/1
  pipeline3/1(q) -> a0p0_1st_shift/6(en)
  pipeline4/1(q) -> fft_biplex/1(sync)
  pipeline5/1(q) -> fft_biplex/2(shift)
  pipeline6/1(q) -> fft_biplex/3(pol00_in)
  pipeline7/1(q) -> fft_biplex/4(pol01_in)
  pipeline8/1(q) -> fft_biplex/5(en)

== system snb_bcxx/pfb_of ==
  out_of0 : Inport
  out_of1 : Inport  Port=2
  assert_of0 : xbsIndex_r4/Assert  assert_type=on  type_source=Explicitly  gui_display_data_type=Fixed-point  arith_type=Unsigned  n_bits=16  bin_pt=0  preci_type=Single  exp_width=8  frac_width=24  assert_rate=off  rate_source=Explicitly  period=1  output_port=on  block_type=assert
  assert_of1 : xbsIndex_r4/Assert  assert_type=on  type_source=Explicitly  gui_display_data_type=Fixed-point  arith_type=Unsigned  n_bits=16  bin_pt=0  preci_type=Single  exp_width=8  frac_width=24  assert_rate=off  rate_source=Explicitly  period=1  output_port=on  block_type=assert
  cast_gw : xbsIndex_r4/Convert  gui_display_data_type=Fixed-point  arith_type=Unsigned  n_bits=32  bin_pt=0  float_type=Single  exp_bits=8  fraction_bits=24  quantization=Truncate  overflow=Wrap  en=off  latency=0  dbl_ovrd=off  pipeline=off  block_type=convert
  concatenate : xbsIndex_r4/Concat  num_inputs=2  dbl_ovrd=off  block_type=concat
  io_delay : xbsIndex_r4/Delay  rst=off  infoeditControl=Selection of Reset will increase slice count due to use of real FFs and instead of SRLs  en=off  latency=0  dbl_ovrd=off  reg_retiming=on  block_type=delay
  reint1 : xbsIndex_r4/Reinterpret  force_arith_type=on  arith_type=Unsigned  force_bin_pt=on  bin_pt=0  block_type=reinterpret
  reint2 : xbsIndex_r4/Reinterpret  force_arith_type=on  arith_type=Unsigned  force_bin_pt=on  bin_pt=0  block_type=reinterpret
  sim_out : Terminator
  snb_bc_pfb_of_user_data_in : xbsIndex_r4/Gateway Out  inherit_from_input=off  hdl_port=on  timing_constraint=None  locs_specified=off  LOCs={}  UseAsDAC=off  DACChannel='1'  block_type=gatewayout
  wires:
  concatenate/1 -> io_delay/1
  io_delay/1 -> cast_gw/1
  cast_gw/1 -> snb_bc_pfb_of_user_data_in/1
  snb_bc_pfb_of_user_data_in/1 -> sim_out/1
  out_of0/1 -> assert_of0/1
  assert_of0/1 -> reint1/1
  reint1/1 -> concatenate/1
  out_of1/1 -> assert_of1/1
  assert_of1/1 -> reint2/1
  reint2/1 -> concatenate/2

== system snb_bcxx/phase_offset0 ==
  sim_1 : Inport
  io_delay : xbsIndex_r4/Delay  rst=off  infoeditControl=Selection of Reset will increase slice count due to use of real FFs and instead of SRLs  en=off  latency=0  dbl_ovrd=off  reg_retiming=on  block_type=delay
  reint1 : xbsIndex_r4/Reinterpret  force_arith_type=on  arith_type=Unsigned  force_bin_pt=on  bin_pt=0  block_type=reinterpret
  slice_phase : xbsIndex_r4/Slice  nbits=32  boolean_output=off  mode=Lower Bit Location + Width  bit1=0  base1=MSB of Input  bit0=0  base0=LSB of Input  dbl_ovrd=off  block_type=slice
  snb_bc_phase_offset0_user_data_out : xbsIndex_r4/Gateway In  gui_display_data_type=Fixed-point  arith_type=Unsigned  n_bits=32  bin_pt=0  preci_type=Single  exp_width=8  frac_width=24  quantization="Round  (unbiased: +/- Inf)"  overflow=Saturate  period=1  dbl_ovrd=off  timing_constraint=None  locs_specified=off  LOCs={}  UseAsADC=off  ADCChannel='1'  inherit_from_input=off  hdl_port=on  block_type=gatewayin
  in_phase : Outport
  wires:
  snb_bc_phase_offset0_user_data_out/1 -> io_delay/1
  sim_1/1 -> snb_bc_phase_offset0_user_data_out/1
  io_delay/1 -> slice_phase/1
  slice_phase/1 -> reint1/1
  reint1/1 -> in_phase/1

== system snb_bcxx/phase_offset1 ==
  sim_1 : Inport
  io_delay : xbsIndex_r4/Delay  rst=off  infoeditControl=Selection of Reset will increase slice count due to use of real FFs and instead of SRLs  en=off  latency=0  dbl_ovrd=off  reg_retiming=on  block_type=delay
  reint1 : xbsIndex_r4/Reinterpret  force_arith_type=on  arith_type=Unsigned  force_bin_pt=on  bin_pt=0  block_type=reinterpret
  slice_phase : xbsIndex_r4/Slice  nbits=32  boolean_output=off  mode=Lower Bit Location + Width  bit1=0  base1=MSB of Input  bit0=0  base0=LSB of Input  dbl_ovrd=off  block_type=slice
  snb_bc_phase_offset1_user_data_out : xbsIndex_r4/Gateway In  gui_display_data_type=Fixed-point  arith_type=Unsigned  n_bits=32  bin_pt=0  preci_type=Single  exp_width=8  frac_width=24  quantization="Round  (unbiased: +/- Inf)"  overflow=Saturate  period=1  dbl_ovrd=off  timing_constraint=None  locs_specified=off  LOCs={}  UseAsADC=off  ADCChannel='1'  inherit_from_input=off  hdl_port=on  block_type=gatewayin
  in_phase : Outport
  wires:
  snb_bc_phase_offset1_user_data_out/1 -> io_delay/1
  sim_1/1 -> snb_bc_phase_offset1_user_data_out/1
  io_delay/1 -> slice_phase/1
  slice_phase/1 -> reint1/1
  reint1/1 -> in_phase/1

== system snb_bcxx/phase_offset_delta0 ==
  sim_1 : Inport
  io_delay : xbsIndex_r4/Delay  rst=off  infoeditControl=Selection of Reset will increase slice count due to use of real FFs and instead of SRLs  en=off  latency=0  dbl_ovrd=off  reg_retiming=on  block_type=delay
  reint1 : xbsIndex_r4/Reinterpret  force_arith_type=on  arith_type=Unsigned  force_bin_pt=on  bin_pt=0  block_type=reinterpret
  slice_phase_offset_delta : xbsIndex_r4/Slice  nbits=32  boolean_output=off  mode=Lower Bit Location + Width  bit1=0  base1=MSB of Input  bit0=0  base0=LSB of Input  dbl_ovrd=off  block_type=slice
  snb_bc_phase_offset_delta0_user_data_out : xbsIndex_r4/Gateway In  gui_display_data_type=Fixed-point  arith_type=Unsigned  n_bits=32  bin_pt=0  preci_type=Single  exp_width=8  frac_width=24  quantization="Round  (unbiased: +/- Inf)"  overflow=Saturate  period=1  dbl_ovrd=off  timing_constraint=None  locs_specified=off  LOCs={}  UseAsADC=off  ADCChannel='1'  inherit_from_input=off  hdl_port=on  block_type=gatewayin
  in_phase_offset_delta : Outport
  wires:
  snb_bc_phase_offset_delta0_user_data_out/1 -> io_delay/1
  sim_1/1 -> snb_bc_phase_offset_delta0_user_data_out/1
  io_delay/1 -> slice_phase_offset_delta/1
  slice_phase_offset_delta/1 -> reint1/1
  reint1/1 -> in_phase_offset_delta/1
